simulink model "axi_stream"  (R2018a)
settings: Solver=VariableStepAuto  StartTime=0.0  StopTime=inf  RelTol=1e-3
undefined symbols (not defined in the file): AXI4, imresize, Lite, rgb2gray
libraries: xbsIndex_r4 x30, simulink x5, hdlsllib x5, dspsrcs4 x1
settings Model: Creator=rgb11127  LastModifiedBy=rgb11127

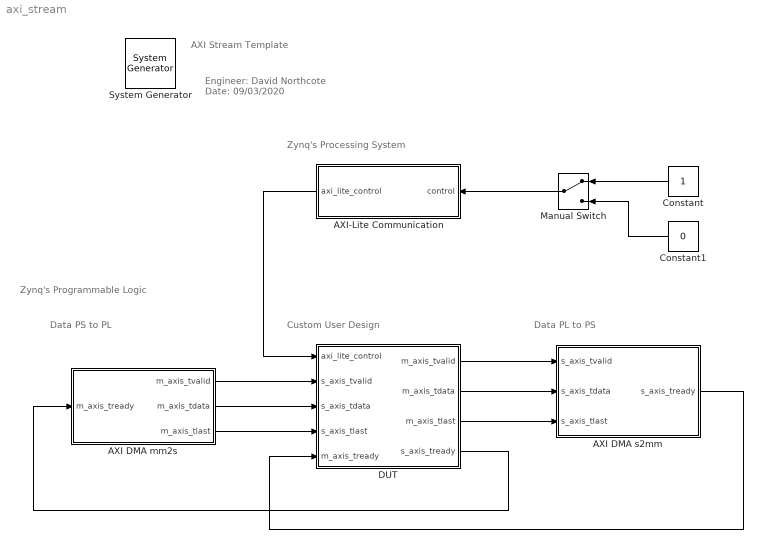
== system axi_stream ==
  note: Zynq's Processing System
  note: Engineer:	David Northcote
      | Date:		09/03/2020
  note: AXI Stream Template
  note: Zynq's Programmable Logic
  note: Data PS to PL
  note: Custom User Design
  note: Data PL to PS
  " System Generator" : xbsIndex_r4/ System Generator  Tag=genX  xilinxfamily=zynq  part=xc7z020  speed=-1  package=clg400  synthesis_tool=Vivado  clock_wrapper=Clock Enables  directory=./netlist  proj_type=Vivado  Synth_file=Vivado Synthesis Defaults  Impl_file=Vivado Implementation Defaults  testbench=off  simulink_period=1/100e6  sysclk_period=10  dcm_input_clock_period=10  incr_netlist=off  trim_vbits=Everywhere in SubSystem  dbl_ovrd=According to Block Masks  core_generation=According to Block Masks  run_coregen=off  deprecated_control=off  eval_field=0  block_type=sysgen
  AXI DMA mm2s : Subsystem  mask{data=rgb2gray(imresize(imread('peppers.png'), [240,320])), rate=1/100e6, bits=8}
      mask prompts: data "Input Data:"; rate "Sample Time:"; bits "Wordlength:"
      mask init:
      | [height, width] = size(data);
      | 
      | totalsize = height*width;
      | 
      | input = reshape(data', [height*width, 1]);
      | 
      | word = str2num(get_param(gcb, 'bits'));
      mask TypeOptions bits: 8 | 16 | 24 | 32 | 40 | 48 | 56 | 64 | 72 | 80 | 88 | 96 | 104 | 112 | 120 | 128
      mask DialogControl DescGroupVar Prompt: AXI DMA mm2s
      mask DialogControl DescTextVar Prompt: This block simulates an AXI-Stream input from an AXI DMA.
      mask DialogControl ParameterGroupVar Prompt: Main
  AXI DMA s2mm : Subsystem  mask{totalsize=240*320, rate=1/100e6}
      mask prompts: totalsize "Buffer Size:"; rate "Sample Rate:"
      mask DialogControl DescGroupVar Prompt: AXI DMA s2mm
      mask DialogControl DescTextVar Prompt: This block simulates an AXI-Stream output to an AXI DMA.
      mask DialogControl ParameterGroupVar Prompt: Main
  AXI-Lite Communication : Subsystem
  Constant : Constant  OutDataTypeStr=uint32  SampleTime=1/100e6
  Constant1 : Constant  Value=0  OutDataTypeStr=uint32  SampleTime=1/100e6
  DUT : Subsystem
  Manual Switch : ManualSwitch
  wires:
  AXI-Lite Communication/1(axi_lite_control) -> DUT/1(axi_lite_control)
  Manual Switch/1 -> AXI-Lite Communication/1(control)
  Constant/1 -> Manual Switch/1
  Constant1/1 -> Manual Switch/2
  AXI DMA mm2s/1(m_axis_tvalid) -> DUT/2(s_axis_tvalid)
  AXI DMA mm2s/2(m_axis_tdata) -> DUT/3(s_axis_tdata)
  AXI DMA mm2s/3(m_axis_tlast) -> DUT/4(s_axis_tlast)
  DUT/1(m_axis_tvalid) -> AXI DMA s2mm/1(s_axis_tvalid)
  DUT/2(m_axis_tdata) -> AXI DMA s2mm/2(s_axis_tdata)
  DUT/3(m_axis_tlast) -> AXI DMA s2mm/3(s_axis_tlast)
  DUT/4(s_axis_tready) -> AXI DMA mm2s/1(m_axis_tready)
  AXI DMA s2mm/1(s_axis_tready) -> DUT/5(m_axis_tready)

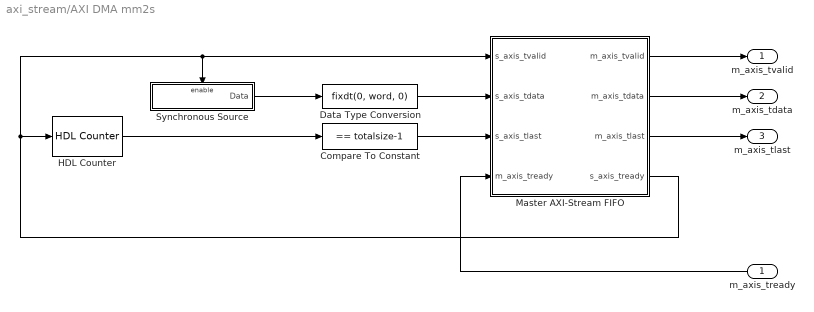
== system axi_stream/AXI DMA mm2s ==
  m_axis_tready : Inport
  Compare To Constant : simulink/Logic and Bit Operations/Compare To Constant  relop===  const=totalsize-1  OutDataTypeStr=boolean
  Data Type Conversion : DataTypeConversion  OutDataTypeStr=fixdt(0, word, 0)  ConvertRealWorld=Stored Integer (SI)
  HDL Counter : hdlsllib/Sources/HDL Counter  CountType=Count limited  CountInit=0  CountStep=1  CountMax=totalsize-1  CountFromType=Initial value  CountFrom=0  CountResetPort=off  CountLoadPort=off  CountEnbPort=on  CountDirPort=off  CountDataType=Unsigned  CountWordLen=ceil(log2(totalsize))  CountFracLen=0  CountSampTime=1
      settings: SourceProductBaseCode=HD
  Master AXI-Stream FIFO : Subsystem  mask{sdepth=32}
      mask prompts: sdepth "FIFO Depth:"
      mask init:
      | set_param([gcb, '/HDL FIFO TDATA'], 'fifo_size', get_param(gcb, 'sdepth'));
      | set_param([gcb, '/HDL FIFO TLAST'], 'fifo_size', get_param(gcb, 'sdepth'));
      | 
      | set_param([gcb, '/Compare To Constant'], 'const', num2str(floor(str2num(get_param(gcb, 'sdepth'))/2)));
      mask TypeOptions sdepth: 16 | 32 | 64 | 128 | 256 | 512 | 1024 | 2048 | 4096 | 8192 | 16384 | 32768
      mask DialogControl DescGroupVar Prompt: Master AXI-Stream FIFO
      mask DialogControl DescTextVar Prompt: A custom AXI-Stream FIFO for sending data to other architectures.
      mask DialogControl ParameterGroupVar Prompt: Main
  Synchronous Source : Subsystem  TreatAsAtomicUnit=on
  m_axis_tvalid : Outport
  m_axis_tdata : Outport  Port=2
  m_axis_tlast : Outport  Port=3
  wires:
  m_axis_tready/1 -> Master AXI-Stream FIFO/4(m_axis_tready)
  Master AXI-Stream FIFO/1(m_axis_tvalid) -> m_axis_tvalid/1
  Master AXI-Stream FIFO/2(m_axis_tdata) -> m_axis_tdata/1
  Master AXI-Stream FIFO/3(m_axis_tlast) -> m_axis_tlast/1
  HDL Counter/1 -> Compare To Constant/1
  Compare To Constant/1 -> Master AXI-Stream FIFO/3(s_axis_tlast)
  Master AXI-Stream FIFO/4(s_axis_tready) -> Synchronous Source/Enable, Master AXI-Stream FIFO/1(s_axis_tvalid), HDL Counter/1
  Synchronous Source/1(Data) -> Data Type Conversion/1
  Data Type Conversion/1 -> Master AXI-Stream FIFO/2(s_axis_tdata)

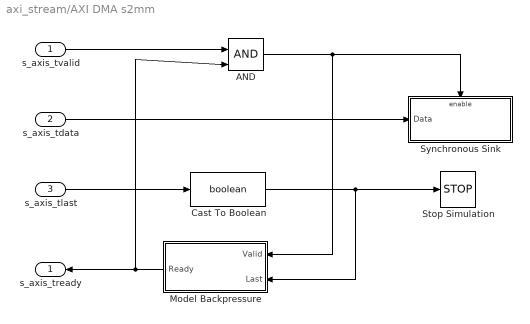
== system axi_stream/AXI DMA s2mm ==
  s_axis_tvalid : Inport
  s_axis_tdata : Inport  Port=2
  s_axis_tlast : Inport  Port=3
  AND : Logic  IconShape=distinctive  AllPortsSameDT=off  OutDataTypeStr=boolean
  Cast To Boolean : DataTypeConversion  OutDataTypeStr=boolean
  Model Backpressure : Subsystem
  Stop Simulation : Stop
  Synchronous Sink : Subsystem  TreatAsAtomicUnit=on
  s_axis_tready : Outport
  wires:
  s_axis_tvalid/1 -> AND/1
  s_axis_tdata/1 -> Synchronous Sink/1(Data)
  s_axis_tlast/1 -> Cast To Boolean/1
  Cast To Boolean/1 -> Model Backpressure/2(Last), Stop Simulation/1
  AND/1 -> Model Backpressure/1(Valid), Synchronous Sink/Enable
  Model Backpressure/1(Ready) -> AND/2, s_axis_tready/1

== system axi_stream/AXI-Lite Communication ==
  control : Inport
  axi_lite_control : Outport
  wires:
  control/1 -> axi_lite_control/1

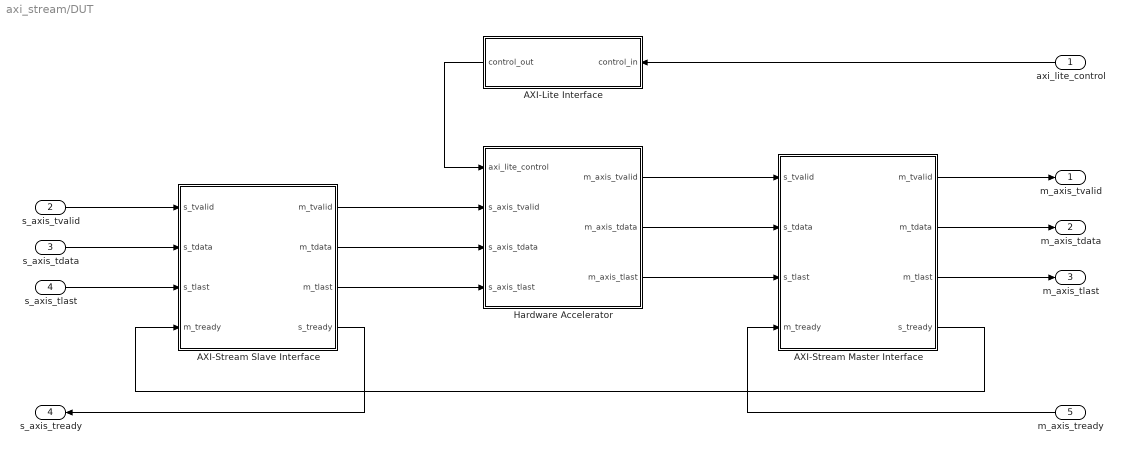
== system axi_stream/DUT ==
  axi_lite_control : Inport
  s_axis_tvalid : Inport  Port=2
  s_axis_tdata : Inport  Port=3
  s_axis_tlast : Inport  Port=4
  m_axis_tready : Inport  Port=5
  AXI-Lite Interface : Subsystem
  AXI-Stream Master Interface : Subsystem  mask{sdepth=16, rate=1/100e6}
      mask prompts: sdepth "FIFO Depth:"; rate "Sample Rate:"
      mask init:
      | set_param([gcb, '/FIFO TLAST'], 'depth', get_param(gcb, 'sdepth')); 
      | set_param([gcb, '/FIFO TDATA'], 'depth', get_param(gcb, 'sdepth')); 
      | 
      | switch get_param(gcb, 'sdepth')
      |     case '16'
      |         depth = 16;
      |     case '32'
      |         depth = 32;
      |     case '64'
      |         depth = 64;
      |     case '128'
      |         depth = 128;
      |     case '256'
      |         depth = 256;
      |     case '512'
      |         depth = 512;
      |     case '1K'
      |         depth = 1024;
      |     case '2K'
      |         depth = 2048;
      |     case '4K'
      |         depth = 4096;
      |     case '8K'
      |         depth = 8192;
      |     case '16K'
      |         depth = 16384;
      |     case '32K'
      |         depth = 32768;
      |     case '64K'
      |         depth = 65536;
      |     case '128K'
      |         depth = 131072;
      |     case '256K'
      |         depth = 262144;
      |     case '512K'
      |         depth = 524288;
      |     case '1M'
      |         depth = 1048576;
      |     case '2M'
      |         depth = 2097152;
      |     case '4M'
      |         depth = 4194304;
      |     otherwise
      |         depth = 16;
      | end
      mask TypeOptions sdepth: 16 | 32 | 64 | 128 | 256 | 512 | 1K | 2K | 4K | 8K | 16K | 32K | 64K | 128K | 256K | 512K | 1M | 2M | 4M
      mask DialogControl DescGroupVar Prompt: AXI-Stream Master Interface
      mask DialogControl DescTextVar Prompt: System generator gateway and FIFO for the AXI-Stream master interface.
      mask DialogControl ParameterGroupVar Prompt: Main
  AXI-Stream Slave Interface : Subsystem  mask{sdepth=16, sbits=8, rate=1/100e6}
      mask prompts: sdepth "FIFO Depth:"; sbits "TData Width:"; rate "Sample Rate:"
      mask init:
      | set_param([gcb, '/FIFO TLAST'], 'depth', get_param(gcb, 'sdepth')); 
      | set_param([gcb, '/FIFO TDATA'], 'depth', get_param(gcb, 'sdepth')); 
      | 
      | bits = str2num(get_param(gcb, 'sbits'));
      mask TypeOptions sdepth: 16 | 32 | 64 | 128 | 256 | 512 | 1K | 2K | 4K | 8K | 16K | 32K | 64K | 128K | 256K | 512K | 1M | 2M | 4M
      mask TypeOptions sbits: 8 | 16 | 24 | 32 | 40 | 48 | 56 | 64 | 72 | 80 | 88 | 96 | 104 | 112 | 120 | 128
      mask DialogControl DescGroupVar Prompt: AXI-Stream Slave Interface
      mask DialogControl DescTextVar Prompt: System generator gateway and FIFO for the AXI-Stream slave interface.
      mask DialogControl ParameterGroupVar Prompt: Main
  Hardware Accelerator : Subsystem
  m_axis_tvalid : Outport
  m_axis_tdata : Outport  Port=2
  m_axis_tlast : Outport  Port=3
  s_axis_tready : Outport  Port=4
  wires:
  s_axis_tvalid/1 -> AXI-Stream Slave Interface/1(s_tvalid)
  s_axis_tdata/1 -> AXI-Stream Slave Interface/2(s_tdata)
  s_axis_tlast/1 -> AXI-Stream Slave Interface/3(s_tlast)
  AXI-Stream Slave Interface/4(s_tready) -> s_axis_tready/1
  AXI-Stream Master Interface/1(m_tvalid) -> m_axis_tvalid/1
  AXI-Stream Master Interface/2(m_tdata) -> m_axis_tdata/1
  AXI-Stream Master Interface/3(m_tlast) -> m_axis_tlast/1
  m_axis_tready/1 -> AXI-Stream Master Interface/4(m_tready)
  Hardware Accelerator/1(m_axis_tvalid) -> AXI-Stream Master Interface/1(s_tvalid)
  Hardware Accelerator/2(m_axis_tdata) -> AXI-Stream Master Interface/2(s_tdata)
  Hardware Accelerator/3(m_axis_tlast) -> AXI-Stream Master Interface/3(s_tlast)
  AXI-Stream Slave Interface/1(m_tvalid) -> Hardware Accelerator/2(s_axis_tvalid)
  AXI-Stream Slave Interface/2(m_tdata) -> Hardware Accelerator/3(s_axis_tdata)
  AXI-Stream Slave Interface/3(m_tlast) -> Hardware Accelerator/4(s_axis_tlast)
  axi_lite_control/1 -> AXI-Lite Interface/1(control_in)
  AXI-Lite Interface/1(control_out) -> Hardware Accelerator/1(axi_lite_control)
  AXI-Stream Master Interface/4(s_tready) -> AXI-Stream Slave Interface/4(m_tready)

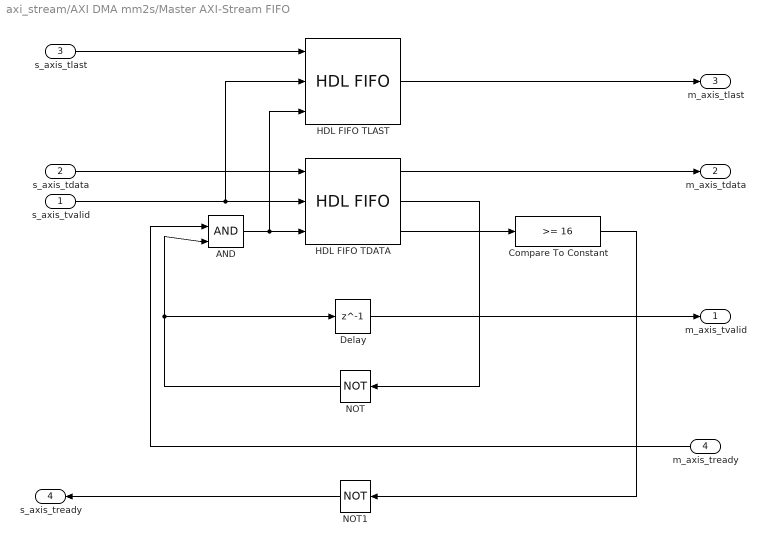
== system axi_stream/AXI DMA mm2s/Master AXI-Stream FIFO ==
  s_axis_tvalid : Inport
  s_axis_tdata : Inport  Port=2
  s_axis_tlast : Inport  Port=3
  m_axis_tready : Inport  Port=4
  AND : Logic  IconShape=distinctive  AllPortsSameDT=off  OutDataTypeStr=boolean
  Compare To Constant : simulink/Logic and Bit Operations/Compare To Constant  relop=>=  const=16  OutDataTypeStr=boolean
  Delay : Delay  DelayLength=1
  HDL FIFO TDATA : hdlsllib/HDL RAMs/HDL FIFO  fifo_size=32  ratio=1  push_msg=Error  pop_msg=Error  show_empty=on  show_full=off  show_num=on
      settings: SourceProductName=HDL Coder  SourceProductBaseCode=HD
  HDL FIFO TLAST : hdlsllib/HDL RAMs/HDL FIFO  fifo_size=32  ratio=1  push_msg=Error  pop_msg=Error  show_empty=off  show_full=off  show_num=off
      settings: SourceProductName=HDL Coder  SourceProductBaseCode=HD
  NOT : Logic  Operator=NOT  IconShape=distinctive  AllPortsSameDT=off  OutDataTypeStr=boolean
  NOT1 : Logic  Operator=NOT  IconShape=distinctive  AllPortsSameDT=off  OutDataTypeStr=boolean
  m_axis_tvalid : Outport
  m_axis_tdata : Outport  Port=2
  m_axis_tlast : Outport  Port=3
  s_axis_tready : Outport  Port=4
  wires:
  HDL FIFO TDATA/3 -> Compare To Constant/1
  Delay/1 -> m_axis_tvalid/1
  s_axis_tlast/1 -> HDL FIFO TLAST/1
  m_axis_tready/1 -> AND/1
  AND/1 -> HDL FIFO TLAST/3, HDL FIFO TDATA/3
  HDL FIFO TDATA/2 -> NOT/1
  NOT/1 -> Delay/1, AND/2
  HDL FIFO TLAST/1 -> m_axis_tlast/1
  HDL FIFO TDATA/1 -> m_axis_tdata/1
  Compare To Constant/1 -> NOT1/1
  NOT1/1 -> s_axis_tready/1
  s_axis_tdata/1 -> HDL FIFO TDATA/1
  s_axis_tvalid/1 -> HDL FIFO TLAST/2, HDL FIFO TDATA/2

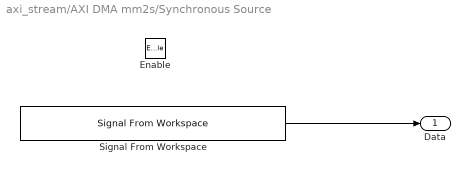
== system axi_stream/AXI DMA mm2s/Synchronous Source ==
  Enable : EnablePort
  Signal From Workspace : dspsrcs4/Signal From Workspace  X=input  Ts=rate  nsamps=1  OutputAfterFinalValue=Setting to zero  ignoreOrWarnInputAndFrameLengths=off  OutputFrames=off
  Data : Outport
  wires:
  Signal From Workspace/1 -> Data/1

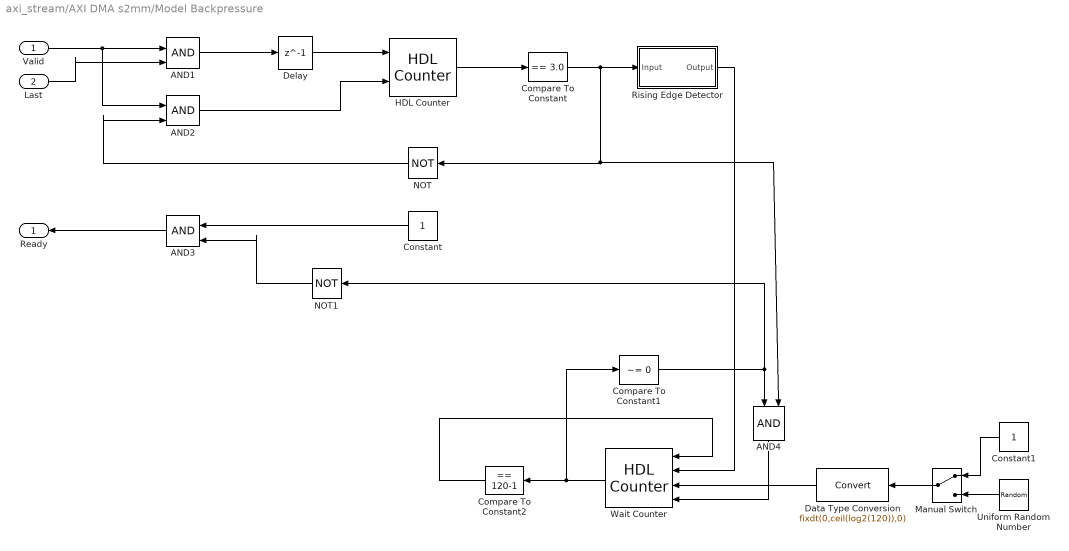
== system axi_stream/AXI DMA s2mm/Model Backpressure ==
  Valid : Inport
  Last : Inport  Port=2
  AND{1..4} (4 alike) : Logic  IconShape=distinctive  AllPortsSameDT=off  OutDataTypeStr=boolean
  Compare To Constant : simulink/Logic and Bit Operations/Compare To Constant  relop===  const=3.0  OutDataTypeStr=boolean
  Compare To Constant1 : simulink/Logic and Bit Operations/Compare To Constant  relop=~=  const=0  OutDataTypeStr=boolean
  Compare To Constant2 : simulink/Logic and Bit Operations/Compare To Constant  relop===  const=120-1  OutDataTypeStr=boolean
  Constant : Constant  OutDataTypeStr=boolean  SampleTime=rate
  Constant1 : Constant  OutDataTypeStr=fixdt(0, ceil(log2(120)), 0)  SampleTime=rate
  Data Type Conversion : DataTypeConversion  OutDataTypeStr=fixdt(0,ceil(log2(120)),0)
  Delay : Delay  DelayLength=1
  HDL Counter : hdlsllib/Sources/HDL Counter  CountType=Count limited  CountInit=0  CountStep=1  CountMax=totalsize-1  CountFromType=Initial value  CountFrom=0  CountResetPort=on  CountLoadPort=off  CountEnbPort=on  CountDirPort=off  CountDataType=Unsigned  CountWordLen=ceil(log2(totalsize))  CountFracLen=0  CountSampTime=1
      settings: SourceProductBaseCode=HD
  Manual Switch : ManualSwitch
  NOT : Logic  Operator=NOT  IconShape=distinctive  AllPortsSameDT=off  OutDataTypeStr=boolean
  NOT1 : Logic  Operator=NOT  IconShape=distinctive  AllPortsSameDT=off  OutDataTypeStr=boolean
  Rising Edge Detector : Subsystem
  Uniform Random Number : UniformRandomNumber  Minimum=0  Maximum=120-1  Seed=round(rand*10)  SampleTime=rate
  Wait Counter : hdlsllib/Sources/HDL Counter  CountType=Count limited  CountInit=0  CountStep=1  CountMax=120-1  CountFromType=Initial value  CountFrom=0  CountResetPort=on  CountLoadPort=on  CountEnbPort=on  CountDirPort=off  CountDataType=Unsigned  CountWordLen=ceil(log2(120))  CountFracLen=0  CountSampTime=1
      settings: SourceProductBaseCode=HD
  Ready : Outport
  wires:
  AND4/1 -> Wait Counter/4
  Constant/1 -> AND3/1
  Data Type Conversion/1 -> Wait Counter/3
  Delay/1 -> HDL Counter/1
  AND1/1 -> Delay/1
  Last/1 -> AND1/2
  Compare To Constant2/1 -> Wait Counter/1
  NOT/1 -> AND2/2
  Compare To Constant1/1 -> NOT1/1, AND4/1
  HDL Counter/1 -> Compare To Constant/1
  Compare To Constant/1 -> AND4/2, NOT/1, Rising Edge Detector/1(Input)
  NOT1/1 -> AND3/2
  Rising Edge Detector/1(Output) -> Wait Counter/2
  Wait Counter/1 -> Compare To Constant2/1, Compare To Constant1/1
  Valid/1 -> AND2/1, AND1/1
  AND2/1 -> HDL Counter/2
  AND3/1 -> Ready/1
  Uniform Random Number/1 -> Manual Switch/2
  Manual Switch/1 -> Data Type Conversion/1
  Constant1/1 -> Manual Switch/1

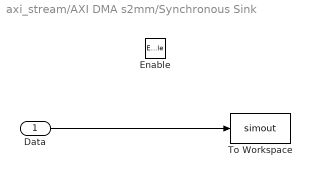
== system axi_stream/AXI DMA s2mm/Synchronous Sink ==
  Data : Inport
  Enable : EnablePort
  To Workspace : ToWorkspace  VariableName=simout  SampleTime=-1
      settings: MaxDataPoints=totalsize  Save2DSignal=2-D array (concatenate along first dimension)
  wires:
  Data/1 -> To Workspace/1

== system axi_stream/DUT/AXI-Lite Interface ==
  control_in : Inport
  ctrl_reg : xbsIndex_r4/Gateway In  gui_display_data_type=Fixed-point  arith_type=Unsigned  n_bits=32  bin_pt=0  preci_type=Single  exp_width=8  frac_width=24  rows=1  columns=1  quantization="Round  (unbiased: +/- Inf)"  overflow=Saturate  period=1/100e6  UseAsADC=off  ADCChannel='1'  interface=AXI4-Lite  automatic_assignment=on  address_offset=hex2dec('00')  intf_name=''  intf_description=''  default_value=0  timing_constraint=None  locs_specified=off  LOCs={}  io_standard={}  inherit_from_input=off  hdl_port=on  dbl_ovrd=off  block_type=gatewayin
  control_out : Outport
  wires:
  control_in/1 -> ctrl_reg/1
  ctrl_reg/1 -> control_out/1

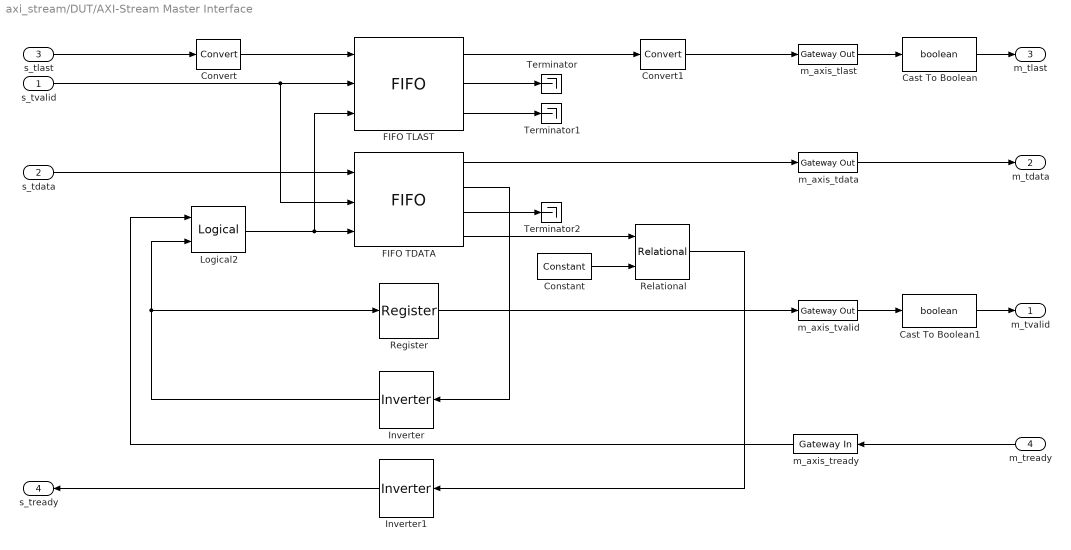
== system axi_stream/DUT/AXI-Stream Master Interface ==
  s_tvalid : Inport
  s_tdata : Inport  Port=2
  s_tlast : Inport  Port=3
  m_tready : Inport  Port=4
  Cast To Boolean : DataTypeConversion  OutDataTypeStr=boolean
  Cast To Boolean1 : DataTypeConversion  OutDataTypeStr=boolean
  Constant : xbsIndex_r4/Constant  const=floor(depth/2)  gui_display_data_type=Fixed-point  arith_type=Unsigned  n_bits=ceil(log2(depth))  bin_pt=0  preci_type=Single  exp_width=8  frac_width=24  explicit_period=on  period=rate  equ=P=C  opselect=C  inp2=PCIN>>17  opr=+  inp1=P  carry=CIN  dbl_ovrd=off  block_type=constant
  Convert : xbsIndex_r4/Convert  gui_display_data_type=Fixed-point  arith_type=Unsigned  n_bits=1  bin_pt=0  float_type=Single  exp_bits=8  fraction_bits=24  quantization=Truncate  overflow=Wrap  en=off  latency=0  pipeline=off  dbl_ovrd=off  block_type=convert
  Convert1 : xbsIndex_r4/Convert  gui_display_data_type=Boolean  arith_type=Boolean  n_bits=1  bin_pt=0  float_type=Single  exp_bits=8  fraction_bits=24  quantization=Truncate  overflow=Wrap  en=off  latency=0  pipeline=off  dbl_ovrd=off  block_type=convert
  FIFO TDATA : xbsIndex_r4/FIFO  mem_type=Distributed RAM  performance_options=Standard_FIFO  embedded_registers=off  depth=16  percent_nbits=1  rst=off  rst_latency=1  en=off  use_dcount=on  use_percent_full_port=off  use_almost_empty=off  almost_empty_thresh=2  use_almost_full=off  almost_full_thresh=14  explicit_period=off  dbl_ovrd=off  block_type=fifo
  FIFO TLAST : xbsIndex_r4/FIFO  mem_type=Distributed RAM  performance_options=Standard_FIFO  embedded_registers=off  depth=16  percent_nbits=1  rst=off  rst_latency=1  en=off  use_dcount=off  use_percent_full_port=off  use_almost_empty=off  almost_empty_thresh=2  use_almost_full=off  almost_full_thresh=14  explicit_period=off  dbl_ovrd=off  block_type=fifo
  Inverter : xbsIndex_r4/Inverter  en=off  latency=0  dbl_ovrd=off  block_type=inv
  Inverter1 : xbsIndex_r4/Inverter  en=off  latency=0  dbl_ovrd=off  block_type=inv
  Logical2 : xbsIndex_r4/Logical  logical_function=AND  inputs=2  en=off  latency=0  precision=Full  arith_type=Unsigned  n_bits=16  bin_pt=0  align_bp=on  dbl_ovrd=off  block_type=logical
  Register : xbsIndex_r4/Register  init=0  rst=off  en=off  dbl_ovrd=off  block_type=register
  Relational : xbsIndex_r4/Relational  mode=a>=b  op_type=Bool  en=off  latency=0  dbl_ovrd=off  block_type=relational
  Terminator : Terminator
  Terminator1 : Terminator
  Terminator2 : Terminator
  m_axis_tdata : xbsIndex_r4/Gateway Out  inherit_from_input=on  hdl_port=on  rows=1  columns=1  UseAsDAC=off  DACChannel='1'  interface=None  automatic_assignment=on  address_offset=hex2dec('00')  intf_name=''  intf_description=''  timing_constraint=None  locs_specified=off  LOCs={}  io_standard={}  block_type=gatewayout
  m_axis_tlast : xbsIndex_r4/Gateway Out  inherit_from_input=on  hdl_port=on  rows=1  columns=1  UseAsDAC=off  DACChannel='1'  interface=None  automatic_assignment=on  address_offset=hex2dec('00')  intf_name=''  intf_description=''  timing_constraint=None  locs_specified=off  LOCs={}  io_standard={}  block_type=gatewayout
  m_axis_tready : xbsIndex_r4/Gateway In  gui_display_data_type=Boolean  arith_type=Boolean  n_bits=16  bin_pt=14  preci_type=Single  exp_width=8  frac_width=24  rows=1  columns=1  quantization="Round  (unbiased: +/- Inf)"  overflow=Saturate  period=rate  UseAsADC=off  ADCChannel='1'  interface=None  automatic_assignment=on  address_offset=hex2dec('00')  intf_name=''  intf_description=''  default_value=0  timing_constraint=None  locs_specified=off  LOCs={}  io_standard={}  inherit_from_input=off  hdl_port=on  dbl_ovrd=off  block_type=gatewayin
  m_axis_tvalid : xbsIndex_r4/Gateway Out  inherit_from_input=on  hdl_port=on  rows=1  columns=1  UseAsDAC=off  DACChannel='1'  interface=None  automatic_assignment=on  address_offset=hex2dec('00')  intf_name=''  intf_description=''  timing_constraint=None  locs_specified=off  LOCs={}  io_standard={}  block_type=gatewayout
  m_tvalid : Outport
  m_tdata : Outport  Port=2
  m_tlast : Outport  Port=3
  s_tready : Outport  Port=4
  wires:
  Inverter1/1 -> s_tready/1
  Convert/1 -> FIFO TLAST/1
  s_tdata/1 -> FIFO TDATA/1
  s_tlast/1 -> Convert/1
  Logical2/1 -> FIFO TLAST/3, FIFO TDATA/3
  m_tready/1 -> m_axis_tready/1
  Inverter/1 -> Register/1, Logical2/2
  FIFO TDATA/2 -> Inverter/1
  FIFO TDATA/1 -> m_axis_tdata/1
  Register/1 -> m_axis_tvalid/1
  FIFO TLAST/1 -> Convert1/1
  FIFO TLAST/3 -> Terminator1/1
  FIFO TLAST/2 -> Terminator/1
  m_axis_tlast/1 -> Cast To Boolean/1
  m_axis_tdata/1 -> m_tdata/1
  m_axis_tvalid/1 -> Cast To Boolean1/1
  m_axis_tready/1 -> Logical2/1
  FIFO TDATA/3 -> Terminator2/1
  FIFO TDATA/4 -> Relational/1
  Constant/1 -> Relational/2
  Relational/1 -> Inverter1/1
  Convert1/1 -> m_axis_tlast/1
  s_tvalid/1 -> FIFO TDATA/2, FIFO TLAST/2
  Cast To Boolean/1 -> m_tlast/1
  Cast To Boolean1/1 -> m_tvalid/1

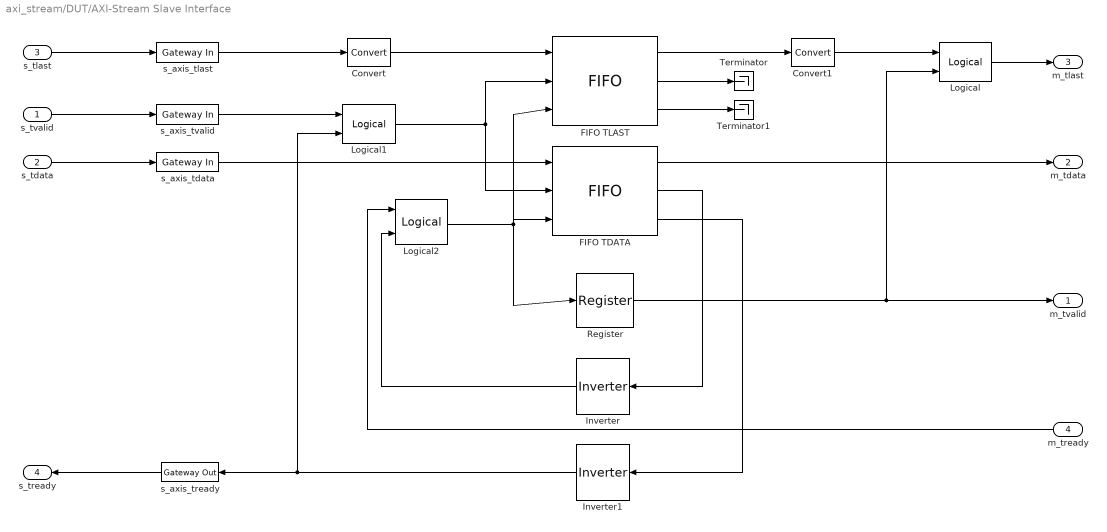
== system axi_stream/DUT/AXI-Stream Slave Interface ==
  s_tvalid : Inport
  s_tdata : Inport  Port=2
  s_tlast : Inport  Port=3
  m_tready : Inport  Port=4
  Convert : xbsIndex_r4/Convert  gui_display_data_type=Fixed-point  arith_type=Unsigned  n_bits=1  bin_pt=0  float_type=Single  exp_bits=8  fraction_bits=24  quantization=Truncate  overflow=Wrap  en=off  latency=0  pipeline=off  dbl_ovrd=off  block_type=convert
  Convert1 : xbsIndex_r4/Convert  gui_display_data_type=Boolean  arith_type=Boolean  n_bits=1  bin_pt=0  float_type=Single  exp_bits=8  fraction_bits=24  quantization=Truncate  overflow=Wrap  en=off  latency=0  pipeline=off  dbl_ovrd=off  block_type=convert
  FIFO TDATA : xbsIndex_r4/FIFO  mem_type=Distributed RAM  performance_options=Standard_FIFO  embedded_registers=off  depth=16  percent_nbits=1  rst=off  rst_latency=1  en=off  use_dcount=off  use_percent_full_port=off  use_almost_empty=off  almost_empty_thresh=2  use_almost_full=off  almost_full_thresh=14  explicit_period=off  dbl_ovrd=off  block_type=fifo
  FIFO TLAST : xbsIndex_r4/FIFO  mem_type=Distributed RAM  performance_options=Standard_FIFO  embedded_registers=off  depth=16  percent_nbits=1  rst=off  rst_latency=1  en=off  use_dcount=off  use_percent_full_port=off  use_almost_empty=off  almost_empty_thresh=2  use_almost_full=off  almost_full_thresh=14  explicit_period=off  dbl_ovrd=off  block_type=fifo
  Inverter : xbsIndex_r4/Inverter  en=off  latency=0  dbl_ovrd=off  block_type=inv
  Inverter1 : xbsIndex_r4/Inverter  en=off  latency=0  dbl_ovrd=off  block_type=inv
  Logical : xbsIndex_r4/Logical  logical_function=AND  inputs=2  en=off  latency=0  precision=Full  arith_type=Unsigned  n_bits=16  bin_pt=0  align_bp=on  dbl_ovrd=off  block_type=logical
  Logical1 : xbsIndex_r4/Logical  logical_function=AND  inputs=2  en=off  latency=0  precision=Full  arith_type=Unsigned  n_bits=16  bin_pt=0  align_bp=on  dbl_ovrd=off  block_type=logical
  Logical2 : xbsIndex_r4/Logical  logical_function=AND  inputs=2  en=off  latency=0  precision=Full  arith_type=Unsigned  n_bits=16  bin_pt=0  align_bp=on  dbl_ovrd=off  block_type=logical
  Register : xbsIndex_r4/Register  init=0  rst=off  en=off  dbl_ovrd=off  block_type=register
  Terminator : Terminator
  Terminator1 : Terminator
  s_axis_tdata : xbsIndex_r4/Gateway In  gui_display_data_type=Fixed-point  arith_type=Unsigned  n_bits=bits  bin_pt=0  preci_type=Single  exp_width=8  frac_width=24  rows=1  columns=1  quantization="Round  (unbiased: +/- Inf)"  overflow=Saturate  period=rate  UseAsADC=off  ADCChannel='1'  interface=None  automatic_assignment=on  address_offset=hex2dec('00')  intf_name=''  intf_description=''  default_value=0  timing_constraint=None  locs_specified=off  LOCs={}  io_standard={}  inherit_from_input=off  hdl_port=on  dbl_ovrd=off  block_type=gatewayin
  s_axis_tlast : xbsIndex_r4/Gateway In  gui_display_data_type=Boolean  arith_type=Boolean  n_bits=16  bin_pt=14  preci_type=Single  exp_width=8  frac_width=24  rows=1  columns=1  quantization="Round  (unbiased: +/- Inf)"  overflow=Saturate  period=rate  UseAsADC=off  ADCChannel='1'  interface=None  automatic_assignment=on  address_offset=hex2dec('00')  intf_name=''  intf_description=''  default_value=0  timing_constraint=None  locs_specified=off  LOCs={}  io_standard={}  inherit_from_input=off  hdl_port=on  dbl_ovrd=off  block_type=gatewayin
  s_axis_tready : xbsIndex_r4/Gateway Out  inherit_from_input=on  hdl_port=on  rows=1  columns=1  UseAsDAC=off  DACChannel='1'  interface=None  automatic_assignment=on  address_offset=hex2dec('00')  intf_name=''  intf_description=''  timing_constraint=None  locs_specified=off  LOCs={}  io_standard={}  block_type=gatewayout
  s_axis_tvalid : xbsIndex_r4/Gateway In  gui_display_data_type=Boolean  arith_type=Boolean  n_bits=16  bin_pt=14  preci_type=Single  exp_width=8  frac_width=24  rows=1  columns=1  quantization="Round  (unbiased: +/- Inf)"  overflow=Saturate  period=rate  UseAsADC=off  ADCChannel='1'  interface=None  automatic_assignment=on  address_offset=hex2dec('00')  intf_name=''  intf_description=''  default_value=0  timing_constraint=None  locs_specified=off  LOCs={}  io_standard={}  inherit_from_input=off  hdl_port=on  dbl_ovrd=off  block_type=gatewayin
  m_tvalid : Outport
  m_tdata : Outport  Port=2
  m_tlast : Outport  Port=3
  s_tready : Outport  Port=4
  wires:
  FIFO TLAST/2 -> Terminator/1
  FIFO TLAST/3 -> Terminator1/1
  FIFO TLAST/1 -> Convert1/1
  Register/1 -> m_tvalid/1, Logical/2
  FIFO TDATA/1 -> m_tdata/1
  Logical/1 -> m_tlast/1
  s_tvalid/1 -> s_axis_tvalid/1
  Logical1/1 -> FIFO TLAST/2, FIFO TDATA/2
  s_tlast/1 -> s_axis_tlast/1
  s_tdata/1 -> s_axis_tdata/1
  FIFO TDATA/2 -> Inverter/1
  FIFO TDATA/3 -> Inverter1/1
  Inverter/1 -> Logical2/2
  m_tready/1 -> Logical2/1
  Inverter1/1 -> Logical1/2, s_axis_tready/1
  Logical2/1 -> Register/1, FIFO TLAST/3, FIFO TDATA/3
  s_axis_tlast/1 -> Convert/1
  s_axis_tvalid/1 -> Logical1/1
  s_axis_tdata/1 -> FIFO TDATA/1
  Convert/1 -> FIFO TLAST/1
  Convert1/1 -> Logical/1
  s_axis_tready/1 -> s_tready/1

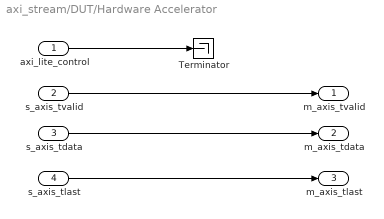
== system axi_stream/DUT/Hardware Accelerator ==
  axi_lite_control : Inport
  s_axis_tvalid : Inport  Port=2
  s_axis_tdata : Inport  Port=3
  s_axis_tlast : Inport  Port=4
  Terminator : Terminator
  m_axis_tvalid : Outport
  m_axis_tdata : Outport  Port=2
  m_axis_tlast : Outport  Port=3
  wires:
  s_axis_tvalid/1 -> m_axis_tvalid/1
  s_axis_tdata/1 -> m_axis_tdata/1
  s_axis_tlast/1 -> m_axis_tlast/1
  axi_lite_control/1 -> Terminator/1

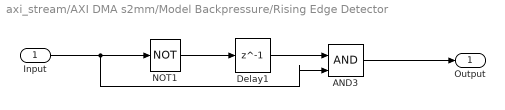
== system axi_stream/AXI DMA s2mm/Model Backpressure/Rising Edge Detector ==
  Input : Inport
  AND3 : Logic  IconShape=distinctive  AllPortsSameDT=off  OutDataTypeStr=boolean
  Delay1 : Delay  DelayLength=1
  NOT1 : Logic  Operator=NOT  IconShape=distinctive  AllPortsSameDT=off  OutDataTypeStr=boolean
  Output : Outport
  wires:
  Input/1 -> AND3/2, NOT1/1
  AND3/1 -> Output/1
  Delay1/1 -> AND3/1
  NOT1/1 -> Delay1/1
